simulink model "lab1_3"  (R2017b)
settings: Solver=VariableStepAuto  StartTime=0.0  StopTime=10.0  RelTol=1e-3
libraries: simulink x1
settings Model: Creator=aseryz  LastModifiedBy=kamzab95
settings CodeAppCC: StateflowObjectComments=on

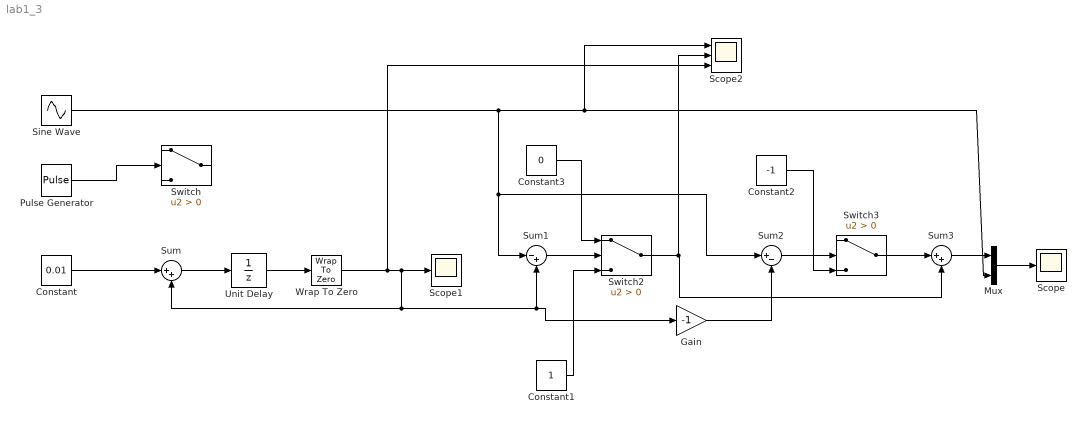
== system lab1_3 ==
  Constant : Constant  Value=0.01
  Constant1 : Constant
  Constant2 : Constant  Value=-1
  Constant3 : Constant  Value=0
  Gain : Gain  Gain=-1
  Mux : Mux  Inputs=2
  Pulse Generator : DiscretePulseGenerator  PulseType=Time based  Period=1  PulseWidth=5
  Scope : Scope
  Scope1 : Scope
  Scope2 : Scope  NumInputPorts=3
  Sine Wave : Sin  SampleTime=0
  Sum : Sum  Inputs=|++
  Sum1 : Sum  Inputs=|-+
  Sum2 : Sum  Inputs=|+-
  Sum3 : Sum  Inputs=|++
  Switch : Switch  Criteria=u2 > Threshold
  Switch2 : Switch  Criteria=u2 > Threshold
  Switch3 : Switch  Criteria=u2 > Threshold
  Unit Delay : UnitDelay  SampleTime=0.001
  Wrap To Zero : simulink/Discontinuities/Wrap To Zero  Threshold=1
      settings: SourceProductName=Simulink  SourceProductBaseCode=SL
  wires:
  Pulse Generator/1 -> Switch/2
  Constant/1 -> Sum/1
  Wrap To Zero/1 -> Scope2/3, Scope1/1, Sum/2, Gain/1, Sum1/2
  Sum1/1 -> Switch2/2
  Constant1/1 -> Switch2/3
  Sine Wave/1 -> Scope2/1, Mux/2, Sum2/1, Sum1/1
  Gain/1 -> Sum2/2
  Sum2/1 -> Switch3/2
  Constant2/1 -> Switch3/3
  Switch2/1 -> Scope2/2, Sum3/2
  Switch3/1 -> Sum3/1
  Sum3/1 -> Mux/1
  Mux/1 -> Scope/1
  Sum/1 -> Unit Delay/1
  Unit Delay/1 -> Wrap To Zero/1
  Constant3/1 -> Switch2/1
